simulink model "Motor_Position_Control_model"  (R2020b)
settings: Solver=VariableStepAuto  StartTime=0.0  StopTime=10.0  RelTol=1e-3
undefined symbols (not defined in the file): b, J, K, Kd, Ki, Kp, L, R
settings Model: Creator=ankit  LastModifiedBy=ankit

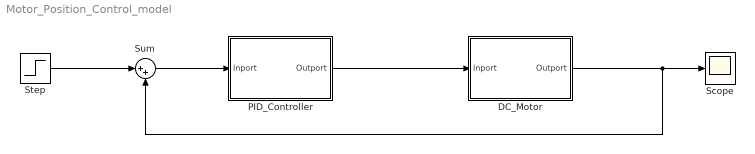
== system Motor_Position_Control_model ==
  DC_Motor : Subsystem
  PID_Controller : Subsystem
  Scope : Scope
  Step : Step  SampleTime=0
  Sum : Sum  Inputs=|++
  wires:
  Step/1 -> Sum/1
  Sum/1 -> PID_Controller/1(Inport)
  PID_Controller/1(Outport) -> DC_Motor/1(Inport)
  DC_Motor/1(Outport) -> Sum/2, Scope/1

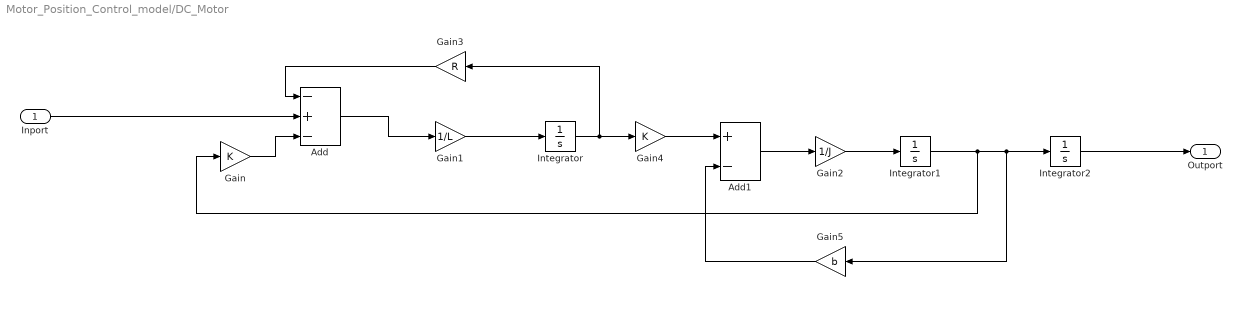
== system Motor_Position_Control_model/DC_Motor ==
  Inport : Inport
  Add : Sum  Inputs=-+-
  Add1 : Sum  Inputs=+-
  Gain : Gain  Gain=K
  Gain1 : Gain  Gain=1/L
  Gain2 : Gain  Gain=1/J
  Gain3 : Gain  Gain=R
  Gain4 : Gain  Gain=K
  Gain5 : Gain  Gain=b
  Integrator : Integrator
  Integrator1 : Integrator
  Integrator2 : Integrator
  Outport : Outport
  wires:
  Add/1 -> Gain1/1
  Inport/1 -> Add/2
  Gain2/1 -> Integrator1/1
  Integrator1/1 -> Gain/1, Gain5/1, Integrator2/1
  Gain3/1 -> Add/1
  Gain4/1 -> Add1/1
  Integrator2/1 -> Outport/1
  Gain/1 -> Add/3
  Add1/1 -> Gain2/1
  Integrator/1 -> Gain4/1, Gain3/1
  Gain1/1 -> Integrator/1
  Gain5/1 -> Add1/2

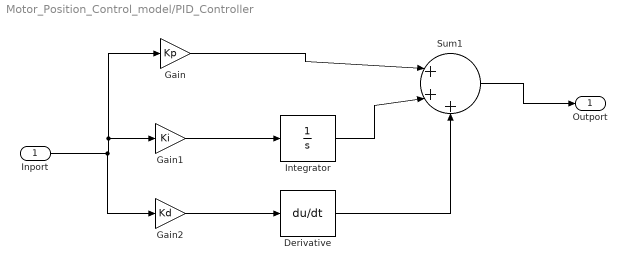
== system Motor_Position_Control_model/PID_Controller ==
  Inport : Inport
  Derivative : Derivative
  Gain : Gain  Gain=Kp
  Gain1 : Gain  Gain=Ki
  Gain2 : Gain  Gain=Kd
  Integrator : Integrator
  Sum1 : Sum  Inputs=|+++
  Outport : Outport
  wires:
  Gain2/1 -> Derivative/1
  Sum1/1 -> Outport/1
  Gain1/1 -> Integrator/1
  Derivative/1 -> Sum1/3
  Gain/1 -> Sum1/1
  Inport/1 -> Gain2/1, Gain1/1, Gain/1
  Integrator/1 -> Sum1/2
